simulink library "INP_BAT"  (R2022a)
settings: Solver=VariableStepAuto  StartTime=0.0  StopTime=10.0  RelTol=1e-3
settings Model: Creator=blatak  LastModifiedBy=blatak

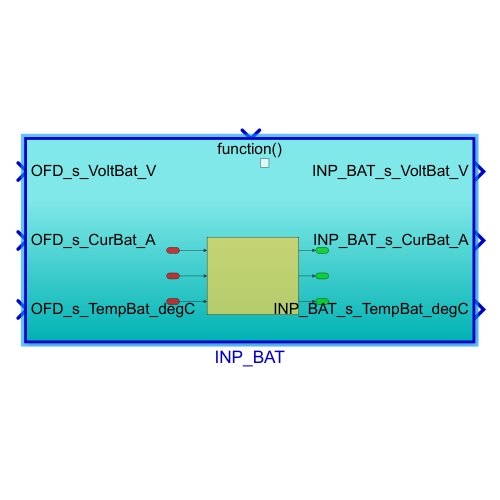
[thumbnail: Simulink's stored preview of the top-level diagram]
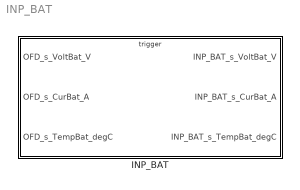
== system INP_BAT ==
  INP_BAT : Subsystem  TreatAsAtomicUnit=on

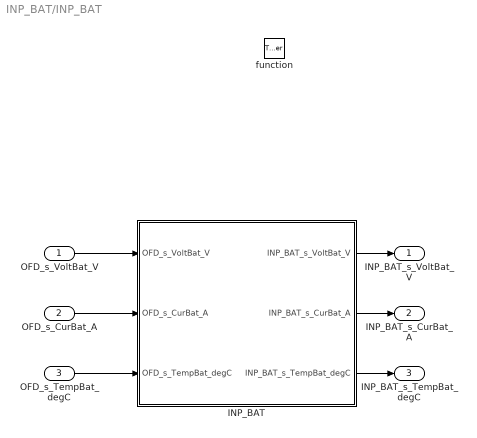
== system INP_BAT/INP_BAT ==
  OFD_s_VoltBat_V : Inport
  OFD_s_CurBat_A : Inport  Port=2
  OFD_s_TempBat_degC : Inport  Port=3
  function : TriggerPort  TriggerType=function-call  VariantControl=(inherit)
  INP_BAT : Subsystem
  INP_BAT_s_VoltBat_V : Outport
  INP_BAT_s_CurBat_A : Outport  Port=2
  INP_BAT_s_TempBat_degC : Outport  Port=3
  wires:
  OFD_s_VoltBat_V/1 -> INP_BAT/1(OFD_s_VoltBat_V)
  OFD_s_CurBat_A/1 -> INP_BAT/2(OFD_s_CurBat_A)
  INP_BAT/1(INP_BAT_s_VoltBat_V) -> INP_BAT_s_VoltBat_V/1
  INP_BAT/2(INP_BAT_s_CurBat_A) -> INP_BAT_s_CurBat_A/1
  OFD_s_TempBat_degC/1 -> INP_BAT/3(OFD_s_TempBat_degC)
  INP_BAT/3(INP_BAT_s_TempBat_degC) -> INP_BAT_s_TempBat_degC/1

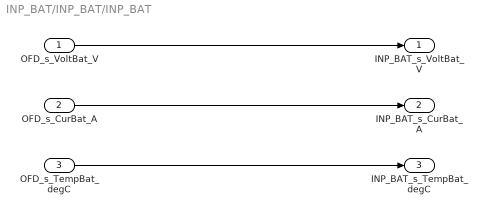
== system INP_BAT/INP_BAT/INP_BAT ==
  OFD_s_VoltBat_V : Inport
  OFD_s_CurBat_A : Inport  Port=2
  OFD_s_TempBat_degC : Inport  Port=3
  INP_BAT_s_VoltBat_V : Outport
  INP_BAT_s_CurBat_A : Outport  Port=2
  INP_BAT_s_TempBat_degC : Outport  Port=3
  wires:
  OFD_s_VoltBat_V/1 -> INP_BAT_s_VoltBat_V/1
  OFD_s_CurBat_A/1 -> INP_BAT_s_CurBat_A/1
  OFD_s_TempBat_degC/1 -> INP_BAT_s_TempBat_degC/1
